simulink model "GM1_Activity_Diagram"  (R2024a)
settings: Solver=VariableStepAuto  StartTime=0.0  StopTime=10.0  RelTol=1e-3
settings Model: Creator=aniru  LastModifiedBy=aniru

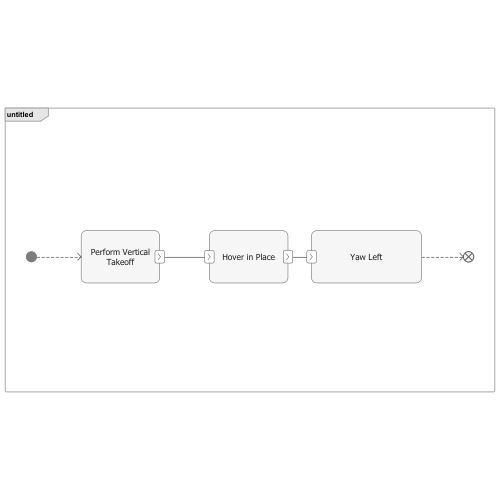
[thumbnail: Simulink's stored preview of the top-level diagram]
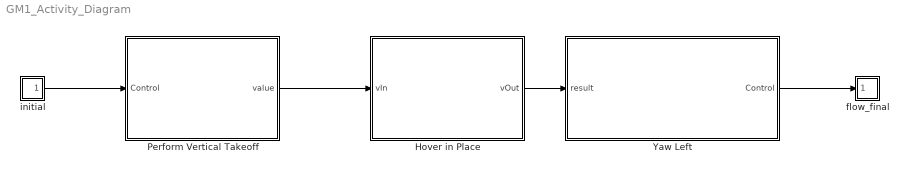
== system GM1_Activity_Diagram ==
  Hover in Place : Subsystem
      settings: CopyFcn=set_param(gcbh,'LinkStatus','none');
  Perform Vertical Takeoff : Subsystem
      settings: CopyFcn=set_param(gcbh,'LinkStatus','none');
  Yaw Left : Subsystem
      settings: CopyFcn=set_param(gcbh,'LinkStatus','none');
  flow_final : Subsystem
      settings: CopyFcn=set_param(gcbh,'LinkStatus','none');
  initial : Subsystem
      settings: CopyFcn=set_param(gcbh,'LinkStatus','none');
  wires:
  initial/1(Control) -> Perform Vertical Takeoff/1(Control)
  Perform Vertical Takeoff/1(value) -> Hover in Place/1(vIn)
  Hover in Place/1(vOut) -> Yaw Left/1(result)
  Yaw Left/1(Control) -> flow_final/1(Control)

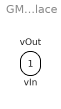
== system GM1_Activity_Diagram/Hover in Place ==
  vIn : Inport
  vOut : Outport

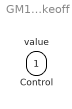
== system GM1_Activity_Diagram/Perform Vertical Takeoff ==
  Control : Inport
  value : Outport

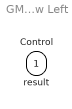
== system GM1_Activity_Diagram/Yaw Left ==
  result : Inport
  Control : Outport

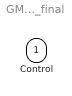
== system GM1_Activity_Diagram/flow_final ==
  Control : Inport

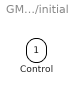
== system GM1_Activity_Diagram/initial ==
  Control : Outport
